simulink model "DC_motor"  (R2025b)
settings: Solver=FixedStepAuto  StartTime=0.0  StopTime=sim_time  FixedStep=dt  MaxStep=dt  RelTol=1e-3
undefined symbols (not defined in the file): b, C, g, Jtot, Kb, Kd, Ki, Kp, Kt, L, m, m_load, R, Vmax, x
libraries: slpidlib x1
settings Model: Creator=gianmarco  LastModifiedBy=gianmarco
settings SolverCC: ZeroCrossControl=EnableAll  EnableFixedStepZeroCrossing=on
settings DataIOCC: SaveFormat=Array

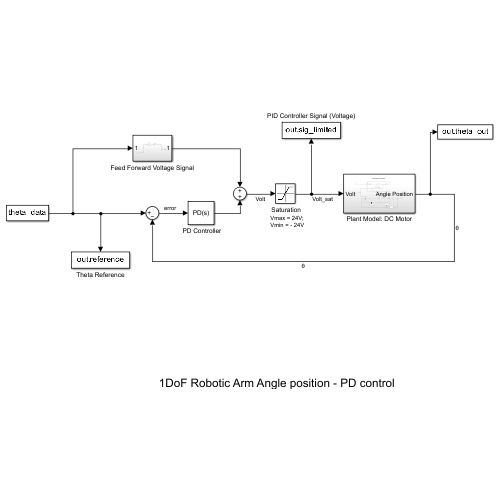
[thumbnail: Simulink's stored preview of the top-level diagram]
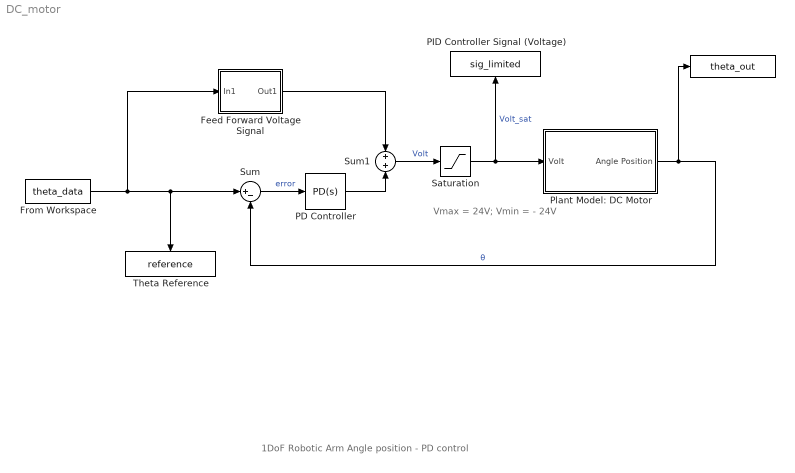
== system DC_motor ==
  note: 1DoF Robotic Arm Angle position - PD control
  note: Vmax = 24V;
      | Vmin = - 24V
  " " : ToWorkspace  VariableName=theta_out  SampleTime=-1
  " PD Controller" : slpidlib/PID Controller  Controller=PD  Form=Parallel  TimeDomain=Continuous-time  UseExternalTs=off  SampleTime=-1  IntegratorMethod=Forward Euler  FilterMethod=Forward Euler  ControllerParametersSource=internal  P=Kp  I=Ki  UseKiTs=off  D=Kd  UseExternalDerivativeSource=off  N=100  UseFilter=on  TunerSelectOption=Transfer Function Based (PID Tuner App)  InitialConditionSource=internal  InitialConditionForIntegrator=0  InitialConditionForFilter=0  DifferentiatorICPrevScaledInput=0  ExternalReset=none  TrackingMode=off  Kt=1  LimitOutput=off  SatLimitsSource=internal  UpperSaturationLimit=inf  LowerSaturationLimit=-inf  LinearizeAsGain=on  AntiWindupMode=none  Kb=1  LimitIntegrator=off  UpperIntegratorSaturationLimit=inf  LowerIntegratorSaturationLimit=-inf  POutMin=[]  POutMax=[]  IOutMin=[]  IOutMax=[]  DOutMin=[]  DOutMax=[]  NOutMin=[]  NOutMax=[]  SumOutMin=[]  SumOutMax=[]  SaturationOutMin=[]  SaturationOutMax=[]  PParamMin=[]  PParamMax=[]  IParamMin=[]  IParamMax=[]  DParamMin=[]  DParamMax=[]  NParamMin=[]  NParamMax=[]  KbParamMin=[]  KbParamMax=[]  KtParamMin=[]  KtParamMax=[]  KbOutMin=[]  KbOutMax=[]  KtOutMin=[]  KtOutMax=[]  IntegratorOutMin=[]  IntegratorOutMax=[]  FilterOutMin=[]  FilterOutMax=[]  SumI1OutMin=[]  SumI1OutMax=[]  SumI2OutMin=[]  SumI2OutMax=[]  SumI3OutMin=[]  SumI3OutMax=[]  SumI4OutMin=[]  SumI4OutMax=[]  SumDOutMin=[]  SumDOutMax=[]  DifferentiatorOutMin=[]  DifferentiatorOutMax=[]  FilterDiffOutCoefMin=[]  FilterDiffOutCoefMax=[]  ReciprocalOutMin=[]  ReciprocalOutMax=[]  SumDenOutMin=[]  SumDenOutMax=[]  SumNumOutMin=[]  SumNumOutMax=[]  DivideOutMin=[]  DivideOutMax=[]  UdiffTsProdOutMin=[]  UdiffTsProdOutMax=[]  NTsProdOutMin=[]  NTsProdOutMax=[]  UintegralTsProdOutMin=[]  UintegralTsProdOutMax=[]  UngainTsProdOutMin=[]  UngainTsProdOutMax=[]  ClampingZeroOutDataTypeStr=Inherit: Inherit via back propagation  ClampingZeroOutMin=[]  ClampingZeroOutMax=[]  FilterDenConstantOutDataTypeStr=Inherit: Inherit via back propagation  FilterDenConstantOutMin=[]  FilterDenConstantOutMax=[]  PCopyOutDataTypeStr=Inherit: Inherit via back propagation  PCopyOutMin=[]  PCopyOutMax=[]  NCopyOutDataTypeStr=Inherit: Inherit via back propagation  NCopyOutMin=[]  NCopyOutMax=[]  IntegratorContinuousStateAttributes=''  IntegratorStateMustResolveToSignalObject=off  IntegratorRTWStateStorageClass=Auto  FilterContinuousStateAttributes=''  FilterStateMustResolveToSignalObject=off  FilterRTWStateStorageClass=Auto  ParallelPVariant=InternalParameters  IdealPVariant=Disabled  IVariant=Disabled  DVariant=InternalParameters  IntegratorVariant=Disabled  SatVariant=Disabled  AWVariant=Disabled  PCopyVariant=Disabled  TRVariant=Disabled  FdbkBlocksVariant=Forward  IdealPFdbkVariant=Disabled  SatFdbkVariant=Disabled  DerivativeFilterVariant=ContFilter  NVariant=InternalParameters  NCopyVariant=Disabled  FilterICVariant=InternalICsFilter  IntegratorICVariant=Disabled  ExternalResetVariant=Disabled  TRSumVariant=Passthrough  SumFdbkVariant=Disabled  SumVariant=Sum_PD  TsampFilterVariant=InternalTs  TsampNgainVariant=Passthrough  TsampIntegralVariant=Disabled_SignalSpec  ExternalSaturationOutDataTypeStr=Inherit: Same as second input  DerivativeSourceVariant=ErrorSignal  PreIntVariant=InternalPreInt
  " Saturation" : Saturate  UpperLimit=Vmax  LowerLimit=-Vmax
  Feed Forward Voltage Signal : Subsystem
  From Workspace : FromWorkspace  VariableName=theta_data
  PID Controller Signal (Voltage) : ToWorkspace  VariableName=sig_limited  SampleTime=-1
  Plant Model: DC Motor : Subsystem
  Sum : Sum  Inputs=|+-
  Sum1 : Sum
  Theta Reference : ToWorkspace  VariableName=reference  SampleTime=-1
  wires:
  Plant Model: DC Motor/1(Angle Position) -> Sum/2, " "/1  "θ"
  Sum/1 -> " PD Controller"/1  "error"
  " Saturation"/1 -> Plant Model: DC Motor/1(Volt), PID Controller Signal (Voltage)/1  "Volt_sat"
  From Workspace/1 -> Feed Forward Voltage Signal/1(In1), Sum/1, Theta Reference/1
  " PD Controller"/1 -> Sum1/2
  Sum1/1 -> " Saturation"/1  "Volt"
  Feed Forward Voltage Signal/1(Out1) -> Sum1/1

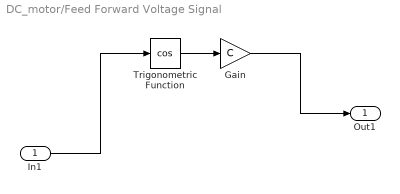
== system DC_motor/Feed Forward Voltage Signal ==
  In1 : Inport
  Gain : Gain  Gain=C
  Trigonometric Function : Trigonometry  Operator=cos
  Out1 : Outport
  wires:
  In1/1 -> Trigonometric Function/1
  Trigonometric Function/1 -> Gain/1
  Gain/1 -> Out1/1

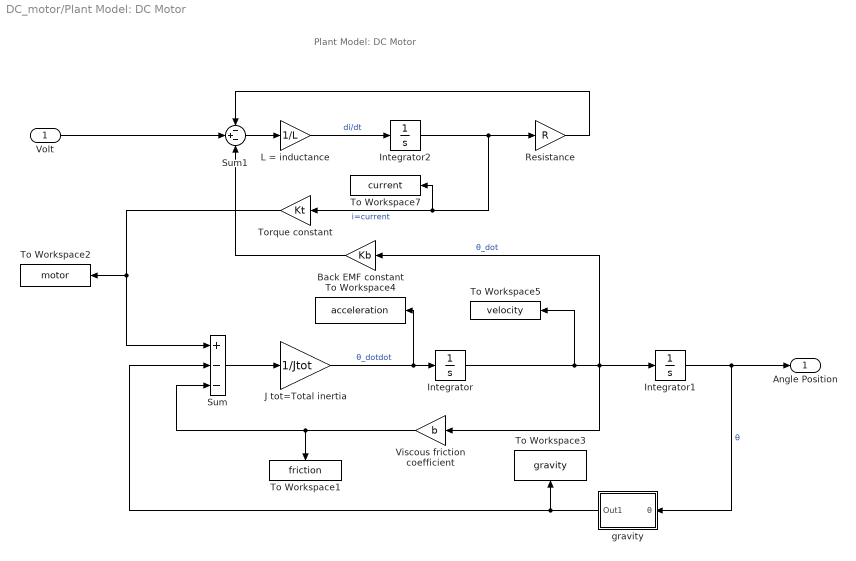
== system DC_motor/Plant Model: DC Motor ==
  note: Plant Model: DC Motor
  Volt : Inport
  "  Integrator" : Integrator
  " Integrator1" : Integrator
  " Resistance" : Gain  Gain=R
  Back EMF constant : Gain  Gain=Kb
  "Integrator2 " : Integrator
  J tot=Total inertia : Gain  Gain=1/Jtot
  L = inductance : Gain  Gain=1/L
  Sum : Sum  Inputs=+--
  Sum1 : Sum  Inputs=-+-
  To Workspace1 : ToWorkspace  VariableName=friction  SampleTime=-1
      settings: Save2DSignal=2-D array (concatenate along first dimension)
  To Workspace2 : ToWorkspace  VariableName=motor  SampleTime=-1
      settings: Save2DSignal=2-D array (concatenate along first dimension)
  To Workspace3 : ToWorkspace  VariableName=gravity  SampleTime=-1
      settings: Save2DSignal=2-D array (concatenate along first dimension)
  To Workspace4 : ToWorkspace  VariableName=acceleration  SampleTime=-1
      settings: Save2DSignal=2-D array (concatenate along first dimension)
  To Workspace5 : ToWorkspace  VariableName=velocity  SampleTime=-1
      settings: Save2DSignal=2-D array (concatenate along first dimension)
  To Workspace7 : ToWorkspace  VariableName=current  SampleTime=-1
      settings: Save2DSignal=2-D array (concatenate along first dimension)
  Torque constant : Gain  Gain=Kt
  Viscous friction coefficient : Gain  Gain=b
  gravity : Subsystem
  Angle Position : Outport
  wires:
  L = inductance/1 -> "Integrator2 "/1  "di/dt"
  " Integrator1"/1 -> Angle Position/1, gravity/1(θ)  "θ"
  Sum/1 -> J tot=Total inertia/1
  "  Integrator"/1 -> To Workspace5/1, Back EMF constant/1, " Integrator1"/1, Viscous friction coefficient/1  "θ_dot"
  Volt/1 -> Sum1/2
  "Integrator2 "/1 -> To Workspace7/1, Torque constant/1, " Resistance"/1  "i=current"
  " Resistance"/1 -> Sum1/1
  Viscous friction coefficient/1 -> Sum/3, To Workspace1/1
  J tot=Total inertia/1 -> "  Integrator"/1, To Workspace4/1  "θ_dotdot"
  Back EMF constant/1 -> Sum1/3
  Sum1/1 -> L = inductance/1
  Torque constant/1 -> Sum/1, To Workspace2/1
  gravity/1(Out1) -> To Workspace3/1, Sum/2

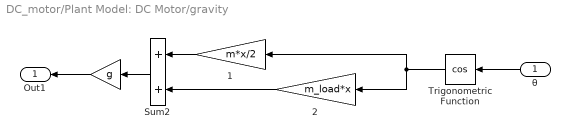
== system DC_motor/Plant Model: DC Motor/gravity ==
  θ : Inport
  " " : Gain  Gain=g
  " 1" : Gain  Gain=m*x/2
  " 2" : Gain  Gain=m_load*x
  Sum2 : Sum
  Trigonometric Function : Trigonometry  Operator=cos
  Out1 : Outport
  wires:
  Trigonometric Function/1 -> " 2"/1, " 1"/1
  " 1"/1 -> Sum2/1
  Sum2/1 -> " "/1
  " 2"/1 -> Sum2/2
  θ/1 -> Trigonometric Function/1
  " "/1 -> Out1/1
